simulink model "pwm_block"  (R2015a)
settings: Solver=ode3  StartTime=0.0  StopTime=3  FixedStep=Ts  RelTol=1e-3
values from neighbouring files (symbols this model uses):
  Tsw = Ts * 10    (= 2e-05)    [VOC_param.m]    (also in power_control_param.m = 0.0002)
settings Model: Creator=rblan  LastModifiedBy=rblan

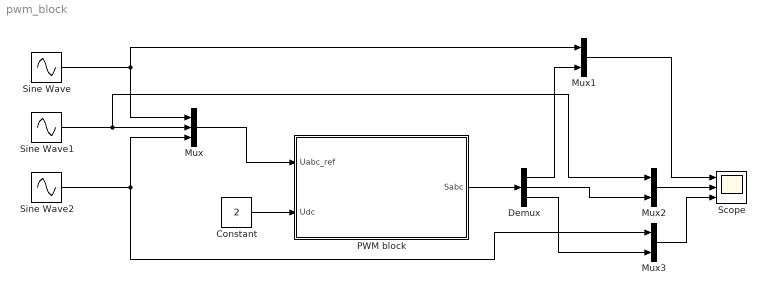
== system pwm_block ==
  Constant : Constant  Value=2
  Demux : Demux  Outputs=3
  Mux : Mux  Inputs=3
  Mux1 : Mux  Inputs=2
  Mux2 : Mux  Inputs=2
  Mux3 : Mux  Inputs=2
  PWM block : Subsystem
  Scope : Scope  NumInputPorts=3
      settings: YMin=-5~-5~-5  YMax=5~5~5
  Sine Wave : Sin  Frequency=50*2*pi  SampleTime=0
  Sine Wave1 : Sin  Frequency=50*2*pi  Phase=2*pi/3  SampleTime=0
  Sine Wave2 : Sin  Frequency=50*2*pi  Phase=4*pi/3  SampleTime=0
  wires:
  Constant/1 -> PWM block/2(Udc)
  Mux/1 -> PWM block/1(Uabc_ref)
  Sine Wave/1 -> Mux/1, Mux1/1
  Sine Wave1/1 -> Mux2/1, Mux/2
  Sine Wave2/1 -> Mux/3, Mux3/1
  Mux1/1 -> Scope/1
  PWM block/1(Sabc) -> Demux/1
  Demux/1 -> Mux1/2
  Mux2/1 -> Scope/2
  Demux/2 -> Mux2/2
  Mux3/1 -> Scope/3
  Demux/3 -> Mux3/2

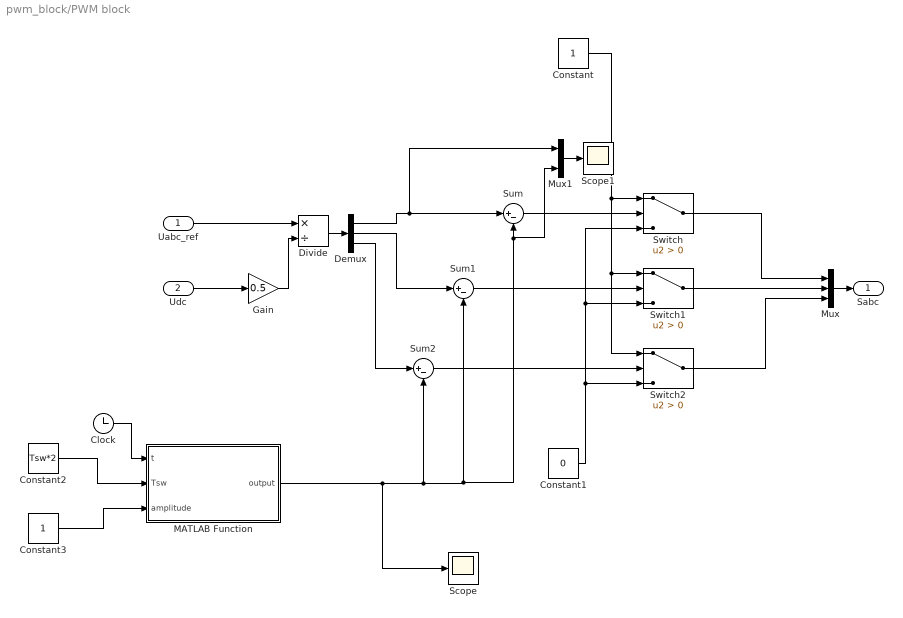
== system pwm_block/PWM block ==
  Uabc_ref : Inport
  Udc : Inport  Port=2
  Clock : Clock
  Constant : Constant
  Constant1 : Constant  Value=0
  Constant2 : Constant  Value=Tsw*2
  Constant3 : Constant
  Demux : Demux  Outputs=3
  Divide : Product  Inputs=*/
  Gain : Gain  Gain=0.5
  MATLAB Function : MATLAB Function  TreatAsAtomicUnit=on
  Mux : Mux  Inputs=3
  Mux1 : Mux  Inputs=2
  Scope : Scope
  Scope1 : Scope
      settings: SaveName=ScopeData2
  Sum : Sum  Inputs=|+-
  Sum1 : Sum  Inputs=|+-
  Sum2 : Sum  Inputs=|+-
  Switch : Switch  Criteria=u2 > Threshold
  Switch1 : Switch  Criteria=u2 > Threshold
  Switch2 : Switch  Criteria=u2 > Threshold
  Sabc : Outport
  wires:
  Mux/1 -> Sabc/1
  Switch/1 -> Mux/1
  Switch1/1 -> Mux/2
  Switch2/1 -> Mux/3
  Constant/1 -> Switch2/1, Switch1/1, Switch/1
  Constant1/1 -> Switch/3, Switch1/3, Switch2/3
  Udc/1 -> Gain/1
  Uabc_ref/1 -> Divide/1
  Gain/1 -> Divide/2
  Divide/1 -> Demux/1
  Demux/1 -> Mux1/1, Sum/1
  Demux/2 -> Sum1/1
  Demux/3 -> Sum2/1
  Sum/1 -> Switch/2
  Sum1/1 -> Switch1/2
  Sum2/1 -> Switch2/2
  MATLAB Function/1(output) -> Scope/1, Mux1/2, Sum/2, Sum1/2, Sum2/2
  Clock/1 -> MATLAB Function/1(t)
  Constant2/1 -> MATLAB Function/2(Tsw)
  Constant3/1 -> MATLAB Function/3(amplitude)
  Mux1/1 -> Scope1/1

== matlab function pwm_block/PWM block/MATLAB Function ==
  data: t input; output output; Tsw input; amplitude input
function output = triangle(t,Tsw,amplitude)
%#codegen
%persistent signal ; 
persistent t_offset ; 

if isempty(t_offset) 
    t_offset = 0 ;  
end

if (t-t_offset>Tsw)
    t_offset = t ; 
    
end 

if ((t-t_offset)<=(Tsw/2))
    signal = -amplitude + (t-t_offset)*2*amplitude/(Tsw/2) ; 
   output = signal ;
   return 


else
    signal = 3*amplitude -  (t-t_offset)*2*amplitude/(Tsw/2) ; 
    output = signal ;
   return 
end 

end
